simulink model "Vehicle_Light"  (R2022b)
settings: Solver=FixedStepAuto  StartTime=0.0  StopTime=100  RelTol=1e-3
model workspace (MAT data in the model file):
  Auto = Simulink.Parameter
  Auto.Value = 1
  Auto.DataType = 'auto'
  Auto.Complexity = 'real'
  Auto.Dimensions = [1 1]
  BehindVehicleDtct = Simulink.Parameter
  BehindVehicleDtct.Value = 3
  BehindVehicleDtct.DataType = 'auto'
  BehindVehicleDtct.Complexity = 'real'
  BehindVehicleDtct.Dimensions = [1 1]
  BrakeLightOff = Simulink.Parameter
  BrakeLightOff.Value = 0
  BrakeLightOff.DataType = 'auto'
  BrakeLightOff.Complexity = 'real'
  BrakeLightOff.Dimensions = [1 1]
  BrakeLightOn = Simulink.Parameter
  BrakeLightOn.Value = 1
  BrakeLightOn.DataType = 'auto'
  BrakeLightOn.Complexity = 'real'
  BrakeLightOn.Dimensions = [1 1]
  BrokeDownPosition = Simulink.Parameter
  BrokeDownPosition.Value = 1
  BrokeDownPosition.DataType = 'auto'
  BrokeDownPosition.Complexity = 'real'
  BrokeDownPosition.Dimensions = [1 1]
  DoorClose = Simulink.Parameter
  DoorClose.Value = 0
  DoorClose.DataType = 'auto'
  DoorClose.Complexity = 'real'
  DoorClose.Dimensions = [1 1]
  DoorOpen = Simulink.Parameter
  DoorOpen.Value = 1
  DoorOpen.DataType = 'auto'
  DoorOpen.Complexity = 'real'
  DoorOpen.Dimensions = [1 1]
  EscortLightOff = Simulink.Parameter
  EscortLightOff.Value = 0
  EscortLightOff.DataType = 'auto'
  EscortLightOff.Complexity = 'real'
  EscortLightOff.Dimensions = [1 1]
  EscortLightOn = Simulink.Parameter
  EscortLightOn.Value = 1
  EscortLightOn.DataType = 'auto'
  EscortLightOn.Complexity = 'real'
  EscortLightOn.Dimensions = [1 1]
  FogDetect = Simulink.Parameter
  FogDetect.Value = 0
  FogDetect.DataType = 'auto'
  FogDetect.Complexity = 'real'
  FogDetect.Dimensions = [1 1]
  HazardLightOff = Simulink.Parameter
  HazardLightOff.Value = 0
  HazardLightOff.DataType = 'auto'
  HazardLightOff.Complexity = 'real'
  HazardLightOff.Dimensions = [1 1]
  HazardLightOn = Simulink.Parameter
  HazardLightOn.Value = 1
  HazardLightOn.DataType = 'auto'
  HazardLightOn.Complexity = 'real'
  HazardLightOn.Dimensions = [1 1]
  HeadLightOff = Simulink.Parameter
  HeadLightOff.Value = 0
  HeadLightOff.DataType = 'auto'
  HeadLightOff.Complexity = 'real'
  HeadLightOff.Dimensions = [1 1]
  HeadLightOn = Simulink.Parameter
  HeadLightOn.Value = 1
  HeadLightOn.DataType = 'auto'
  HeadLightOn.Complexity = 'real'
  HeadLightOn.Dimensions = [1 1]
  HighBeam = Simulink.Parameter
  HighBeam.Value = 2
  HighBeam.DataType = 'auto'
  HighBeam.Complexity = 'real'
  HighBeam.Dimensions = [1 1]
  Highway = Simulink.Parameter
  Highway.Value = 1
  Highway.DataType = 'auto'
  Highway.Complexity = 'real'
  Highway.Dimensions = [1 1]
  Ignition_OFF = Simulink.Parameter
  Ignition_OFF.Value = 0
  Ignition_OFF.DataType = 'auto'
  Ignition_OFF.Complexity = 'real'
  Ignition_OFF.Dimensions = [1 1]
  Ignition_ON = Simulink.Parameter
  Ignition_ON.Value = 1
  Ignition_ON.DataType = 'auto'
  Ignition_ON.Complexity = 'real'
  Ignition_ON.Dimensions = [1 1]
  InsideCity = Simulink.Parameter
  InsideCity.Value = 4
  InsideCity.DataType = 'auto'
  InsideCity.Complexity = 'real'
  InsideCity.Dimensions = [1 1]
  LeftIndicator = Simulink.Parameter
  LeftIndicator.Value = 2
  LeftIndicator.DataType = 'auto'
  LeftIndicator.Complexity = 'real'
  LeftIndicator.Dimensions = [1 1]
  LeftSideAngle = Simulink.Parameter
  LeftSideAngle.Value = -10
  LeftSideAngle.DataType = 'auto'
  LeftSideAngle.Complexity = 'real'
  LeftSideAngle.Dimensions = [1 1]
  LowBeam = Simulink.Parameter
  LowBeam.Value = 3
  LowBeam.DataType = 'auto'
  LowBeam.Complexity = 'real'
  LowBeam.Dimensions = [1 1]
  LuggageCompartmentClose = Simulink.Parameter
  LuggageCompartmentClose.Value = 0
  LuggageCompartmentClose.DataType = 'auto'
  LuggageCompartmentClose.Complexity = 'real'
  LuggageCompartmentClose.Dimensions = [1 1]
  LuggageCompartmentOpen = Simulink.Parameter
  LuggageCompartmentOpen.Value = 1
  LuggageCompartmentOpen.DataType = 'auto'
  LuggageCompartmentOpen.Complexity = 'real'
  LuggageCompartmentOpen.Dimensions = [1 1]
  Manual = Simulink.Parameter
  Manual.Value = 0
  Manual.DataType = 'auto'
  Manual.Complexity = 'real'
  Manual.Dimensions = [1 1]
  NoVehicleDtct = Simulink.Parameter
  NoVehicleDtct.Value = 0
  NoVehicleDtct.DataType = 'auto'
  NoVehicleDtct.Complexity = 'real'
  NoVehicleDtct.Dimensions = [1 1]
  OnComingVehicle = Simulink.Parameter
  OnComingVehicle.Value = 2
  OnComingVehicle.DataType = 'auto'
  OnComingVehicle.Complexity = 'real'
  OnComingVehicle.Dimensions = [1 1]
  OutsideCity = Simulink.Parameter
  OutsideCity.Value = 2
  OutsideCity.DataType = 'auto'
  OutsideCity.Complexity = 'real'
  OutsideCity.Dimensions = [1 1]
  RainDetect = Simulink.Parameter
  RainDetect.Value = 1
  RainDetect.DataType = 'auto'
  RainDetect.Complexity = 'real'
  RainDetect.Dimensions = [1 1]
  ReadingLightOff = Simulink.Parameter
  ReadingLightOff.Value = 0
  ReadingLightOff.DataType = 'auto'
  ReadingLightOff.Complexity = 'real'
  ReadingLightOff.Dimensions = [1 1]
  ReadingLightOn = Simulink.Parameter
  ReadingLightOn.Value = 1
  ReadingLightOn.DataType = 'auto'
  ReadingLightOn.Complexity = 'real'
  ReadingLightOn.Dimensions = [1 1]
  RightIndicator = Simulink.Parameter
  RightIndicator.Value = 1
  RightIndicator.DataType = 'auto'
  RightIndicator.Complexity = 'real'
  RightIndicator.Dimensions = [1 1]
  RightSideAngle = Simulink.Parameter
  RightSideAngle.Value = 10
  RightSideAngle.DataType = 'auto'
  RightSideAngle.Complexity = 'real'
  RightSideAngle.Dimensions = [1 1]
  SpdLmt = Simulink.Parameter
  SpdLmt.Value = 40
  SpdLmt.DataType = 'auto'
  SpdLmt.Complexity = 'real'
  SpdLmt.Dimensions = [1 1]
  StationaryPosition = Simulink.Parameter
  StationaryPosition.Value = 0
  StationaryPosition.DataType = 'auto'
  StationaryPosition.Complexity = 'real'
  StationaryPosition.Dimensions = [1 1]
  TailLightOff = Simulink.Parameter
  TailLightOff.Value = 3
  TailLightOff.DataType = 'auto'
  TailLightOff.Complexity = 'real'
  TailLightOff.Dimensions = [1 1]
  TailLightOn = Simulink.Parameter
  TailLightOn.Value = 2
  TailLightOn.DataType = 'auto'
  TailLightOn.Complexity = 'real'
  TailLightOn.Dimensions = [1 1]
  Tunnel = Simulink.Parameter
  Tunnel.Value = 3
  Tunnel.DataType = 'auto'
  Tunnel.Complexity = 'real'
  Tunnel.Dimensions = [1 1]
  VehicleDtct = Simulink.Parameter
  VehicleDtct.Value = 1
  VehicleDtct.DataType = 'auto'
  VehicleDtct.Complexity = 'real'
  VehicleDtct.Dimensions = [1 1]
  VehicleLck = Simulink.Parameter
  VehicleLck.Value = 1
  VehicleLck.DataType = 'auto'
  VehicleLck.Complexity = 'real'
  VehicleLck.Dimensions = [1 1]
  VehicleSpd = Simulink.Parameter
  VehicleSpd.Value = 80
  VehicleSpd.DataType = 'auto'
  VehicleSpd.Complexity = 'real'
  VehicleSpd.Dimensions = [1 1]
  VehicleUnlck = Simulink.Parameter
  VehicleUnlck.Value = 0
  VehicleUnlck.DataType = 'auto'
  VehicleUnlck.Complexity = 'real'
  VehicleUnlck.Dimensions = [1 1]
undefined symbols (not defined in the file): BehindVeh_Detect, Fog_Detect, LightSystem, NoVeh_Detect, Rain_Detect, VehicleSpeed
libraries: simulink x74
settings Model: DataDictionary=test.sldd  Creator=sanke  LastModifiedBy=Shaileja Swami
settings DebuggingCC: ParameterPrecisionLossMsg=none  UnconnectedInputMsg=warning  UnconnectedOutputMsg=warning  UnconnectedLineMsg=warning
settings ModelReferenceCC: EnableRefExpFcnMdlSchedulingChecks=on
settings RTWCC: DLArmComputeVersion=19.05

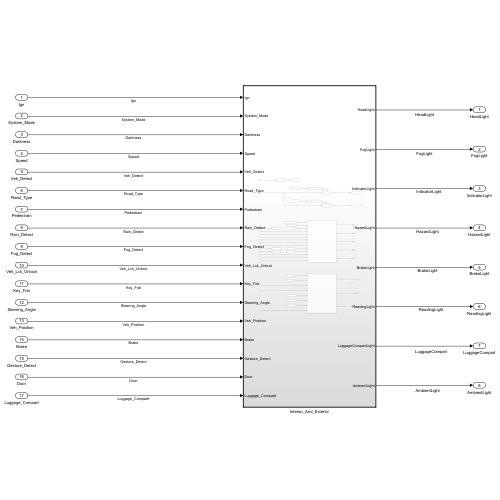
[thumbnail: Simulink's stored preview of the top-level diagram]
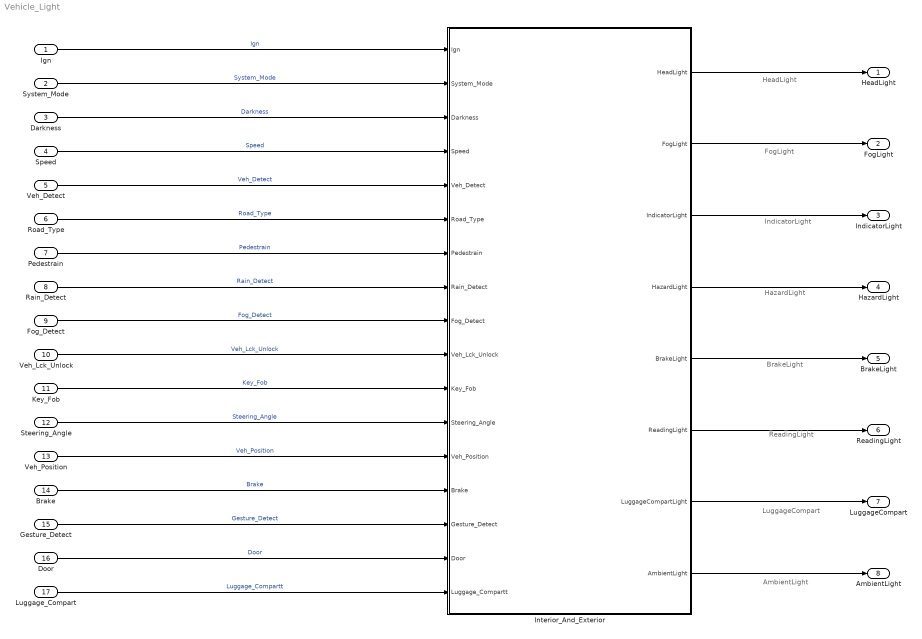
== system Vehicle_Light ==
  note: AmbientLight
  note: LuggageCompart
  note: ReadingLight
  note: BrakeLight
  note: HazardLight
  note: IndicatorLight
  note: FogLight
  note: HeadLight
  Ign : Inport
  System_Mode : Inport  Port=2
  Darkness : Inport  Port=3
  Speed : Inport  Port=4
  Veh_Detect : Inport  Port=5
  Road_Type : Inport  Port=6
  Pedestrain : Inport  Port=7
  Rain_Detect : Inport  Port=8
  Fog_Detect : Inport  Port=9
  Veh_Lck_Unlock : Inport  Port=10
  Key_Fob : Inport  Port=11
  Steering_Angle : Inport  Port=12
  Veh_Position : Inport  Port=13
  Brake : Inport  Port=14
  Gesture_Detect : Inport  Port=15
  Door : Inport  Port=16
  Luggage_Compart : Inport  Port=17
  Interior_And_Exterior : Subsystem  TreatAsAtomicUnit=on
  HeadLight : Outport
  FogLight : Outport  Port=2
  IndicatorLight : Outport  Port=3
  HazardLight : Outport  Port=4
  BrakeLight : Outport  Port=5
  ReadingLight : Outport  Port=6
  LuggageCompart : Outport  Port=7
  AmbientLight : Outport  Port=8
  wires:
  Ign/1 -> Interior_And_Exterior/1(Ign)  "Ign"
  Veh_Detect/1 -> Interior_And_Exterior/5(Veh_Detect)  "Veh_Detect"
  Brake/1 -> Interior_And_Exterior/14(Brake)  "Brake"
  Key_Fob/1 -> Interior_And_Exterior/11(Key_Fob)  "Key_Fob"
  Fog_Detect/1 -> Interior_And_Exterior/9(Fog_Detect)  "Fog_Detect"
  Interior_And_Exterior/8(AmbientLight) -> AmbientLight/1
  Steering_Angle/1 -> Interior_And_Exterior/12(Steering_Angle)  "Steering_Angle"
  Road_Type/1 -> Interior_And_Exterior/6(Road_Type)  "Road_Type"
  Speed/1 -> Interior_And_Exterior/4(Speed)  "Speed"
  Interior_And_Exterior/4(HazardLight) -> HazardLight/1
  Pedestrain/1 -> Interior_And_Exterior/7(Pedestrain)  "Pedestrain"
  Rain_Detect/1 -> Interior_And_Exterior/8(Rain_Detect)  "Rain_Detect"
  Veh_Lck_Unlock/1 -> Interior_And_Exterior/10(Veh_Lck_Unlock)  "Veh_Lck_Unlock"
  Luggage_Compart/1 -> Interior_And_Exterior/17(Luggage_Compartt)  "Luggage_Compartt"
  System_Mode/1 -> Interior_And_Exterior/2(System_Mode)  "System_Mode"
  Interior_And_Exterior/5(BrakeLight) -> BrakeLight/1
  Interior_And_Exterior/2(FogLight) -> FogLight/1
  Interior_And_Exterior/6(ReadingLight) -> ReadingLight/1
  Veh_Position/1 -> Interior_And_Exterior/13(Veh_Position)  "Veh_Position"
  Door/1 -> Interior_And_Exterior/16(Door)  "Door"
  Interior_And_Exterior/7(LuggageCompartLight) -> LuggageCompart/1
  Interior_And_Exterior/1(HeadLight) -> HeadLight/1
  Darkness/1 -> Interior_And_Exterior/3(Darkness)  "Darkness"
  Interior_And_Exterior/3(IndicatorLight) -> IndicatorLight/1
  Gesture_Detect/1 -> Interior_And_Exterior/15(Gesture_Detect)  "Gesture_Detect"

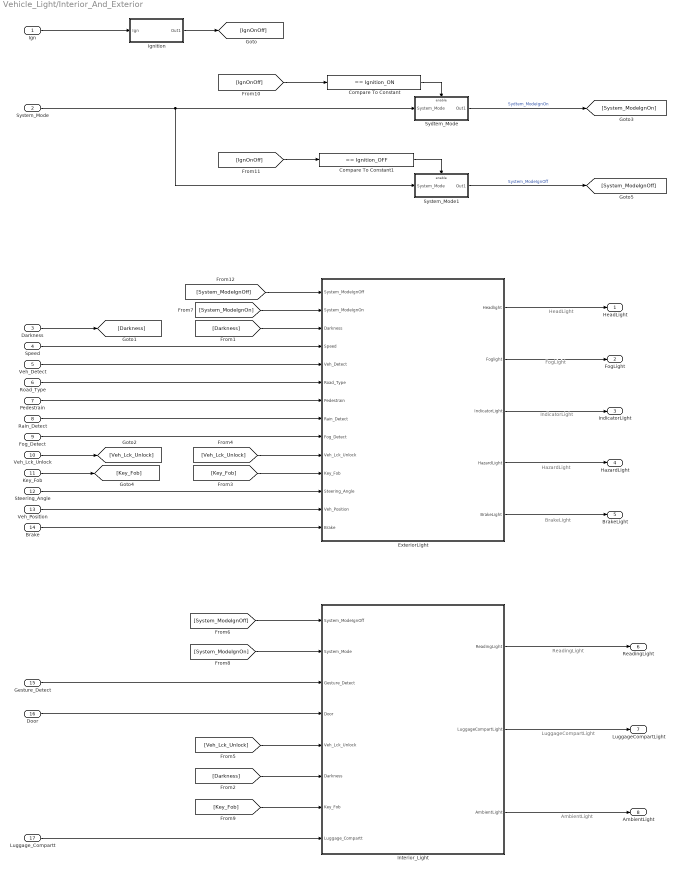
== system Vehicle_Light/Interior_And_Exterior ==
  note: HeadLight
  note: FogLight
  note: IndicatorLight
  note: HazardLight
  note: BrakeLight
  note: ReadingLight
  note: LuggageCompartLight
  note: AmbientLight
  Ign : Inport
  System_Mode : Inport  Port=2
  Darkness : Inport  Port=3
  Speed : Inport  Port=4
  Veh_Detect : Inport  Port=5
  Road_Type : Inport  Port=6
  Pedestrain : Inport  Port=7
  Rain_Detect : Inport  Port=8
  Fog_Detect : Inport  Port=9
  Veh_Lck_Unlock : Inport  Port=10
  Key_Fob : Inport  Port=11
  Steering_Angle : Inport  Port=12
  Veh_Position : Inport  Port=13
  Brake : Inport  Port=14
  Gesture_Detect : Inport  Port=15
  Door : Inport  Port=16
  Luggage_Compartt : Inport  Port=17
  Compare To Constant : simulink/Logic and Bit Operations/Compare To Constant  relop===  const=Ignition_ON  OutDataTypeStr=boolean
  Compare To Constant1 : simulink/Logic and Bit Operations/Compare To Constant  relop===  const=Ignition_OFF  OutDataTypeStr=boolean
  ExteriorLight : Subsystem  TreatAsAtomicUnit=on
  Ignition : Subsystem  TreatAsAtomicUnit=on
  Interior_Light : Subsystem  TreatAsAtomicUnit=on
  Sydtem_Mode : Subsystem  TreatAsAtomicUnit=on
  System_Mode1 : Subsystem  TreatAsAtomicUnit=on
  HeadLight : Outport
  FogLight : Outport  Port=2
  IndicatorLight : Outport  Port=3
  HazardLight : Outport  Port=4
  BrakeLight : Outport  Port=5
  ReadingLight : Outport  Port=6
  LuggageCompartLight : Outport  Port=7
  AmbientLight : Outport  Port=8
  wires:
  Ign/1 -> Ignition/1(Ign)
  System_Mode/1 -> Sydtem_Mode/1(System_Mode), System_Mode1/1(System_Mode)
  Ignition/1(Out1) -> [IgnOnOff]
  [System_ModeIgnOff] -> ExteriorLight/1(System_ModeIgnOff)
  Speed/1 -> ExteriorLight/4(Speed)
  Veh_Detect/1 -> ExteriorLight/5(Veh_Detect)
  Road_Type/1 -> ExteriorLight/6(Road_Type)
  Pedestrain/1 -> ExteriorLight/7(Pedestrain)
  Rain_Detect/1 -> ExteriorLight/8(Rain_Detect)
  Fog_Detect/1 -> ExteriorLight/9(Fog_Detect)
  Steering_Angle/1 -> ExteriorLight/12(Steering_Angle)
  Veh_Position/1 -> ExteriorLight/13(Veh_Position)
  Brake/1 -> ExteriorLight/14(Brake)
  ExteriorLight/1(Headlight) -> HeadLight/1
  ExteriorLight/2(Foglight) -> FogLight/1
  ExteriorLight/3(IndicatorLight) -> IndicatorLight/1
  ExteriorLight/4(HazardLight) -> HazardLight/1
  ExteriorLight/5(BrakeLight) -> BrakeLight/1
  Gesture_Detect/1 -> Interior_Light/3(Gesture_Detect)
  Door/1 -> Interior_Light/4(Door)
  Luggage_Compartt/1 -> Interior_Light/8(Luggage_Compartt)
  Darkness/1 -> [Darkness]
  [Darkness] -> ExteriorLight/3(Darkness)
  [Darkness] -> Interior_Light/6(Darkness)
  Veh_Lck_Unlock/1 -> [Veh_Lck_Unlock]
  [Veh_Lck_Unlock] -> ExteriorLight/10(Veh_Lck_Unlock)
  [Veh_Lck_Unlock] -> Interior_Light/5(Veh_Lck_Unlock)
  Interior_Light/1(ReadingLight) -> ReadingLight/1
  Interior_Light/2(LuggageCompartLight) -> LuggageCompartLight/1
  [System_ModeIgnOff] -> Interior_Light/1(System_ModeIgnOff)
  Sydtem_Mode/1(Out1) -> [System_ModeIgnOn]  "Sydtem_ModeIgnOn"
  [System_ModeIgnOn] -> ExteriorLight/2(System_ModeIgnOn)
  [System_ModeIgnOn] -> Interior_Light/2(System_Mode)
  Interior_Light/3(AmbientLight) -> AmbientLight/1
  Key_Fob/1 -> [Key_Fob]
  [Key_Fob] -> ExteriorLight/11(Key_Fob)
  [Key_Fob] -> Interior_Light/7(Key_Fob)
  [IgnOnOff] -> Compare To Constant/1
  [IgnOnOff] -> Compare To Constant1/1
  Compare To Constant/1 -> Sydtem_Mode/Enable
  Compare To Constant1/1 -> System_Mode1/Enable
  System_Mode1/1(Out1) -> [System_ModeIgnOff]  "System_ModeIgnOff"

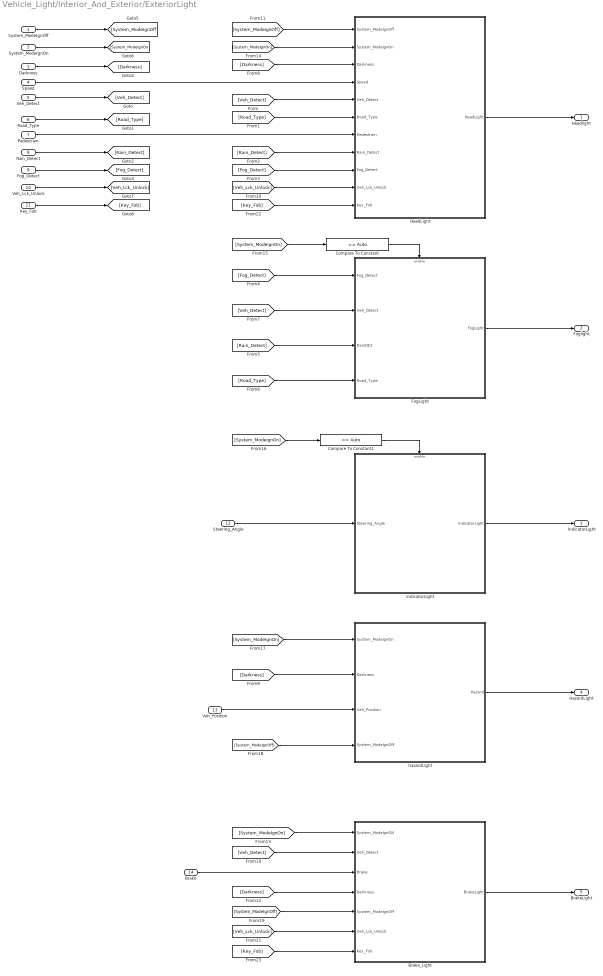
== system Vehicle_Light/Interior_And_Exterior/ExteriorLight ==
  System_ModeIgnOff : Inport
  System_ModeIgnOn : Inport  Port=2
  Darkness : Inport  Port=3
  Speed : Inport  Port=4
  Veh_Detect : Inport  Port=5
  Road_Type : Inport  Port=6
  Pedestrain : Inport  Port=7
  Rain_Detect : Inport  Port=8
  Fog_Detect : Inport  Port=9
  Veh_Lck_Unlock : Inport  Port=10
  Key_Fob : Inport  Port=11
  Steering_Angle : Inport  Port=12
  Veh_Position : Inport  Port=13
  Brake : Inport  Port=14
  Brake_Light : Subsystem  TreatAsAtomicUnit=on
  Compare To Constant : simulink/Logic and Bit Operations/Compare To Constant  relop===  const=Auto  OutDataTypeStr=boolean
  Compare To Constant1 : simulink/Logic and Bit Operations/Compare To Constant  relop===  const=Auto  OutDataTypeStr=boolean
  FogLight : Subsystem  TreatAsAtomicUnit=on
  HeadLight : Subsystem  TreatAsAtomicUnit=on
  hazardLight : Subsystem  TreatAsAtomicUnit=on
  indicatorLight : Subsystem  TreatAsAtomicUnit=on
  Headlight : Outport
  Foglight : Outport  Port=2
  IndicatorLight : Outport  Port=3
  HazardLight : Outport  Port=4
  BrakeLight : Outport  Port=5
  wires:
  Speed/1 -> HeadLight/4(Speed)
  Pedestrain/1 -> HeadLight/7(Pedestrain)
  Veh_Detect/1 -> [Veh_Detect]
  Road_Type/1 -> [Road_Type]
  Rain_Detect/1 -> [Rain_Detect]
  Fog_Detect/1 -> [Fog_Detect]
  [Veh_Detect] -> HeadLight/5(Veh_Detect)
  [Road_Type] -> HeadLight/6(Road_Type)
  [Rain_Detect] -> HeadLight/8(Rain_Detect)
  [Fog_Detect] -> HeadLight/9(Fog_Detect)
  [Fog_Detect] -> FogLight/1(Fog_Detect)
  [Rain_Detect] -> FogLight/3(RainDtct)
  [Road_Type] -> FogLight/4(Road_Type)
  [Veh_Detect] -> FogLight/2(Veh_Detect)
  Steering_Angle/1 -> indicatorLight/1(Steering_Angle)
  Darkness/1 -> [Darkness]
  [Darkness] -> HeadLight/3(Darkness)
  [Darkness] -> hazardLight/2(Darkness)
  Veh_Position/1 -> hazardLight/3(Veh_Position)
  [Veh_Detect] -> Brake_Light/2(Veh_Detect)
  Brake/1 -> Brake_Light/3(Brake)
  FogLight/1(FogLight) -> Foglight/1
  indicatorLight/1(IndicatorLight) -> IndicatorLight/1
  [Darkness] -> Brake_Light/4(Darkness)
  System_ModeIgnOff/1 -> [System_ModeIgnOff]
  [System_ModeIgnOff] -> HeadLight/1(System_ModeIgnOff)
  [System_ModeIgnOff] -> Brake_Light/5(System_ModeIgnOff)
  HeadLight/1(HeadLight) -> Headlight/1
  System_ModeIgnOn/1 -> [System_ModeIgnOn]
  [System_ModeIgnOn] -> HeadLight/2(System_ModeIgnOn)
  [System_ModeIgnOn] -> Compare To Constant/1
  Compare To Constant/1 -> FogLight/Enable
  [System_ModeIgnOn] -> Compare To Constant1/1
  Compare To Constant1/1 -> indicatorLight/Enable
  [System_ModeIgnOff] -> hazardLight/4(System_ModeIgnOff)
  [System_ModeIgnOn] -> hazardLight/1(System_ModeIgnOn)
  hazardLight/1(Hazard) -> HazardLight/1
  [System_ModeIgnOn] -> Brake_Light/1(System_ModeIgnON)
  Veh_Lck_Unlock/1 -> [Veh_Lck_Unlock]
  [Veh_Lck_Unlock] -> HeadLight/10(Veh_Lck_Unlock)
  [Veh_Lck_Unlock] -> Brake_Light/6(Veh_Lck_Unlock)
  Key_Fob/1 -> [Key_Fob]
  [Key_Fob] -> HeadLight/11(Key_Fob)
  [Key_Fob] -> Brake_Light/7(Key_Fob)
  Brake_Light/1(BrakeLight) -> BrakeLight/1

== system Vehicle_Light/Interior_And_Exterior/Ignition ==
  Ign : Inport
  Constant : Constant  Value=Ignition_ON  SampleTime=-1
  Constant1 : Constant  Value=Ignition_OFF  SampleTime=-1
  Switch : Switch  Criteria=u2 > Threshold  SaturateOnIntegerOverflow=off  InputSameDT=off
  Out1 : Outport
  wires:
  Ign/1 -> Switch/2
  Switch/1 -> Out1/1
  Constant/1 -> Switch/1
  Constant1/1 -> Switch/3

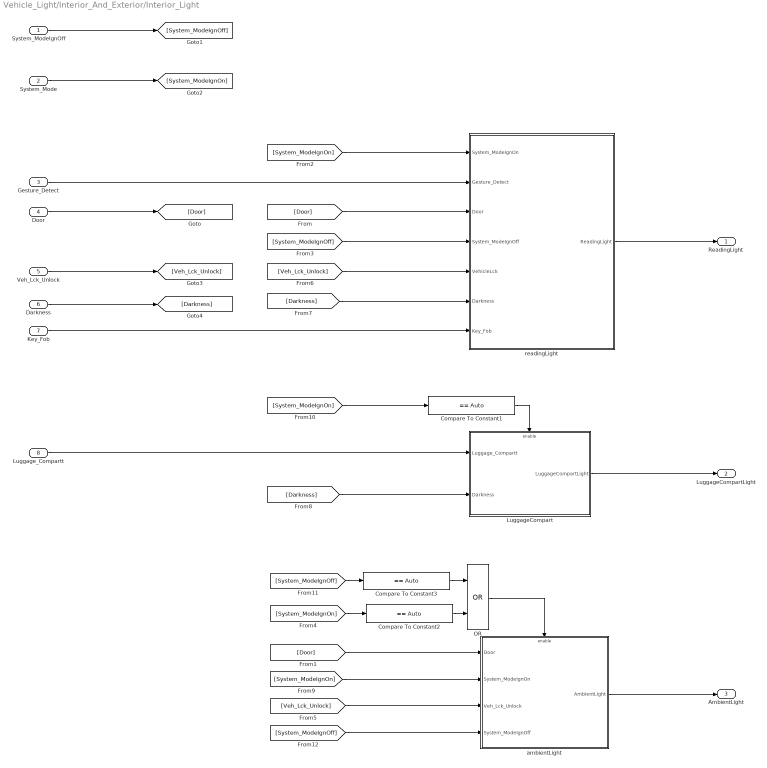
== system Vehicle_Light/Interior_And_Exterior/Interior_Light ==
  System_ModeIgnOff : Inport
  System_Mode : Inport  Port=2
  Gesture_Detect : Inport  Port=3
  Door : Inport  Port=4
  Veh_Lck_Unlock : Inport  Port=5
  Darkness : Inport  Port=6
  Key_Fob : Inport  Port=7
  Luggage_Compartt : Inport  Port=8
  Compare To Constant1 : simulink/Logic and Bit Operations/Compare To Constant  relop===  const=Auto  OutDataTypeStr=boolean
  Compare To Constant2 : simulink/Logic and Bit Operations/Compare To Constant  relop===  const=Auto  OutDataTypeStr=boolean
  Compare To Constant3 : simulink/Logic and Bit Operations/Compare To Constant  relop===  const=Auto  OutDataTypeStr=boolean
  LuggageCompart : Subsystem  TreatAsAtomicUnit=on
  OR : Logic  Operator=OR  AllPortsSameDT=off  OutDataTypeStr=boolean
  ambientLight : Subsystem  TreatAsAtomicUnit=on
  readingLight : Subsystem  TreatAsAtomicUnit=on
  ReadingLight : Outport
  LuggageCompartLight : Outport  Port=2
  AmbientLight : Outport  Port=3
  wires:
  Gesture_Detect/1 -> readingLight/2(Gesture_Detect)
  Luggage_Compartt/1 -> LuggageCompart/1(Luggage_Compartt)
  LuggageCompart/1(LuggageCompartLight) -> LuggageCompartLight/1
  Door/1 -> [Door]
  [Door] -> readingLight/3(Door)
  [Door] -> ambientLight/1(Door)
  ambientLight/1(AmbientLight) -> AmbientLight/1
  System_ModeIgnOff/1 -> [System_ModeIgnOff]
  [System_ModeIgnOn] -> readingLight/1(System_ModeIgnOn)
  [System_ModeIgnOff] -> readingLight/4(System_ModeIgnOff)
  Veh_Lck_Unlock/1 -> [Veh_Lck_Unlock]
  [Veh_Lck_Unlock] -> ambientLight/3(Veh_Lck_Unlock)
  [Veh_Lck_Unlock] -> readingLight/5(VehicleLck)
  Darkness/1 -> [Darkness]
  [Darkness] -> readingLight/6(Darkness)
  [Darkness] -> LuggageCompart/2(Darkness)
  [System_ModeIgnOn] -> ambientLight/2(System_ModeIgnOn)
  Compare To Constant1/1 -> LuggageCompart/Enable
  [System_ModeIgnOn] -> Compare To Constant1/1
  Key_Fob/1 -> readingLight/7(Key_Fob)
  System_Mode/1 -> [System_ModeIgnOn]
  [System_ModeIgnOn] -> Compare To Constant2/1
  readingLight/1(ReadingLight) -> ReadingLight/1
  [System_ModeIgnOff] -> Compare To Constant3/1
  Compare To Constant3/1 -> OR/1
  Compare To Constant2/1 -> OR/2
  OR/1 -> ambientLight/Enable
  [System_ModeIgnOff] -> ambientLight/4(System_ModeIgnOff)

== system Vehicle_Light/Interior_And_Exterior/Sydtem_Mode ==
  System_Mode : Inport
  Enable : EnablePort
  Constant : Constant  Value=Auto  SampleTime=-1
  Constant1 : Constant  Value=Manual  SampleTime=-1
  Switch : Switch  Criteria=u2 > Threshold  SaturateOnIntegerOverflow=off  InputSameDT=off
  Out1 : Outport
  wires:
  Switch/1 -> Out1/1
  System_Mode/1 -> Switch/2
  Constant/1 -> Switch/1
  Constant1/1 -> Switch/3

== system Vehicle_Light/Interior_And_Exterior/System_Mode1 ==
  System_Mode : Inport
  Enable : EnablePort
  Constant : Constant  Value=Auto  SampleTime=-1
  Constant1 : Constant  Value=Manual  SampleTime=-1
  Switch : Switch  Criteria=u2 > Threshold  SaturateOnIntegerOverflow=off  InputSameDT=off
  Out1 : Outport
  wires:
  Constant1/1 -> Switch/3
  Constant/1 -> Switch/1
  System_Mode/1 -> Switch/2
  Switch/1 -> Out1/1

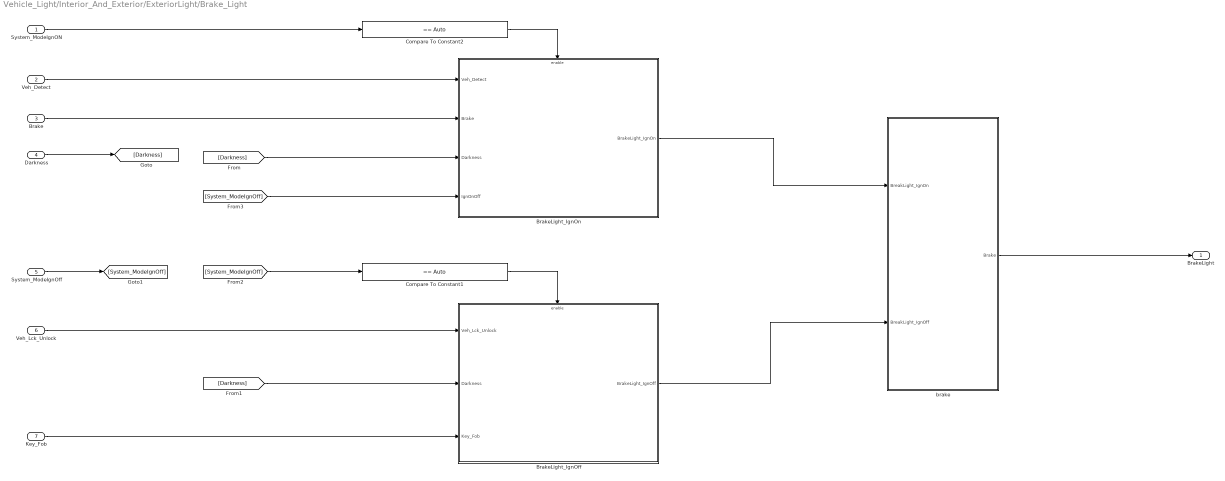
== system Vehicle_Light/Interior_And_Exterior/ExteriorLight/Brake_Light ==
  System_ModeIgnON : Inport
  Veh_Detect : Inport  Port=2
  Brake : Inport  Port=3
  Darkness : Inport  Port=4
  System_ModeIgnOff : Inport  Port=5
  Veh_Lck_Unlock : Inport  Port=6
  Key_Fob : Inport  Port=7
  BrakeLight_IgnOff : Subsystem
  BrakeLight_IgnOn : Subsystem
  Compare To Constant1 : simulink/Logic and Bit Operations/Compare To Constant  relop===  const=Auto  OutDataTypeStr=boolean
  Compare To Constant2 : simulink/Logic and Bit Operations/Compare To Constant  relop===  const=Auto  OutDataTypeStr=boolean
  brake : Subsystem
  BrakeLight : Outport
  wires:
  Veh_Detect/1 -> BrakeLight_IgnOn/1(Veh_Detect)
  Brake/1 -> BrakeLight_IgnOn/2(Brake)
  Darkness/1 -> [Darkness]
  [Darkness] -> BrakeLight_IgnOn/3(Darkness)
  [Darkness] -> BrakeLight_IgnOff/2(Darkness)
  Veh_Lck_Unlock/1 -> BrakeLight_IgnOff/1(Veh_Lck_Unlock)
  Key_Fob/1 -> BrakeLight_IgnOff/3(Key_Fob)
  Compare To Constant1/1 -> BrakeLight_IgnOff/Enable
  System_ModeIgnOff/1 -> [System_ModeIgnOff]
  [System_ModeIgnOff] -> Compare To Constant1/1
  [System_ModeIgnOff] -> BrakeLight_IgnOn/4(IgnOnOff)
  Compare To Constant2/1 -> BrakeLight_IgnOn/Enable
  System_ModeIgnON/1 -> Compare To Constant2/1
  BrakeLight_IgnOff/1(BrakeLight_IgnOff) -> brake/2(BreakLight_IgnOff)
  BrakeLight_IgnOn/1(BrakeLight_IgnOn) -> brake/1(BreakLight_IgnOn)
  brake/1(Brake) -> BrakeLight/1

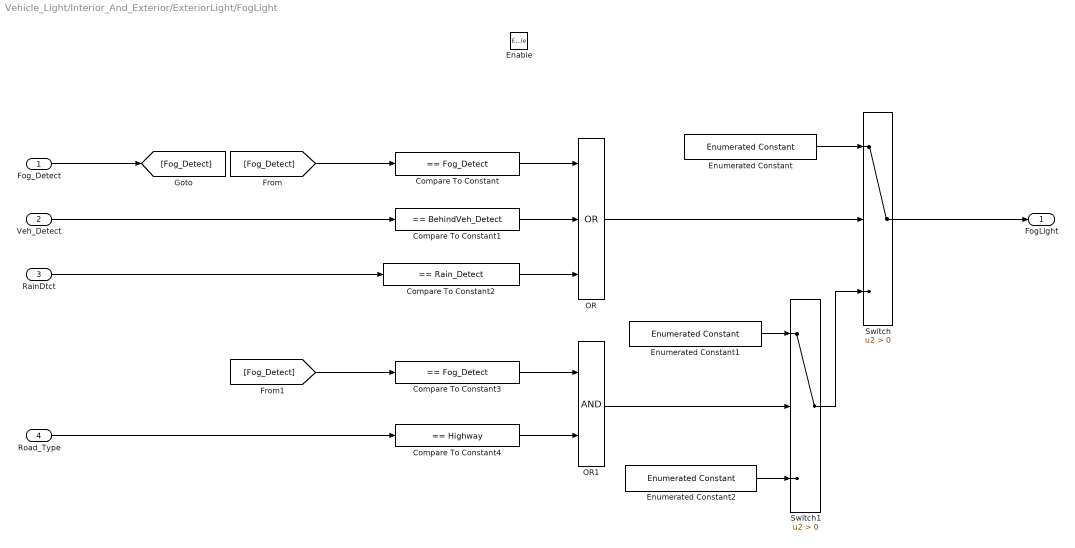
== system Vehicle_Light/Interior_And_Exterior/ExteriorLight/FogLight ==
  Fog_Detect : Inport
  Veh_Detect : Inport  Port=2
  RainDtct : Inport  Port=3
  Road_Type : Inport  Port=4
  Enable : EnablePort
  Compare To Constant : simulink/Logic and Bit Operations/Compare To Constant  relop===  const=Fog_Detect  OutDataTypeStr=boolean
  Compare To Constant1 : simulink/Logic and Bit Operations/Compare To Constant  relop===  const=BehindVeh_Detect  OutDataTypeStr=boolean
  Compare To Constant2 : simulink/Logic and Bit Operations/Compare To Constant  relop===  const=Rain_Detect  OutDataTypeStr=boolean
  Compare To Constant3 : simulink/Logic and Bit Operations/Compare To Constant  relop===  const=Fog_Detect  OutDataTypeStr=boolean
  Compare To Constant4 : simulink/Logic and Bit Operations/Compare To Constant  relop===  const=Highway  OutDataTypeStr=boolean
  Enumerated Constant : simulink/Sources/Enumerated Constant  OutDataTypeStr=Enum: LightSystem  Value=LightSystem.FogLightOn  SampleTime=-1
  Enumerated Constant1 : simulink/Sources/Enumerated Constant  OutDataTypeStr=Enum: LightSystem  Value=LightSystem.FogLightOff  SampleTime=-1
  Enumerated Constant2 : simulink/Sources/Enumerated Constant  OutDataTypeStr=Enum: LightSystem  Value=LightSystem.FogLightOff  SampleTime=-1
  OR : Logic  Operator=OR  Inputs=3  AllPortsSameDT=off  OutDataTypeStr=boolean
  OR1 : Logic  AllPortsSameDT=off  OutDataTypeStr=boolean
  Switch : Switch  Criteria=u2 > Threshold  SaturateOnIntegerOverflow=off  InputSameDT=off
  Switch1 : Switch  Criteria=u2 > Threshold  SaturateOnIntegerOverflow=off  InputSameDT=off
  FogLight : Outport
  wires:
  Switch1/1 -> Switch/3
  OR/1 -> Switch/2
  OR1/1 -> Switch1/2
  Compare To Constant/1 -> OR/1
  Compare To Constant1/1 -> OR/2
  Compare To Constant2/1 -> OR/3
  Compare To Constant3/1 -> OR1/1
  Compare To Constant4/1 -> OR1/2
  Veh_Detect/1 -> Compare To Constant1/1
  RainDtct/1 -> Compare To Constant2/1
  Road_Type/1 -> Compare To Constant4/1
  Fog_Detect/1 -> [Fog_Detect]
  [Fog_Detect] -> Compare To Constant/1
  [Fog_Detect] -> Compare To Constant3/1
  Switch/1 -> FogLight/1
  Enumerated Constant/1 -> Switch/1
  Enumerated Constant1/1 -> Switch1/1
  Enumerated Constant2/1 -> Switch1/3

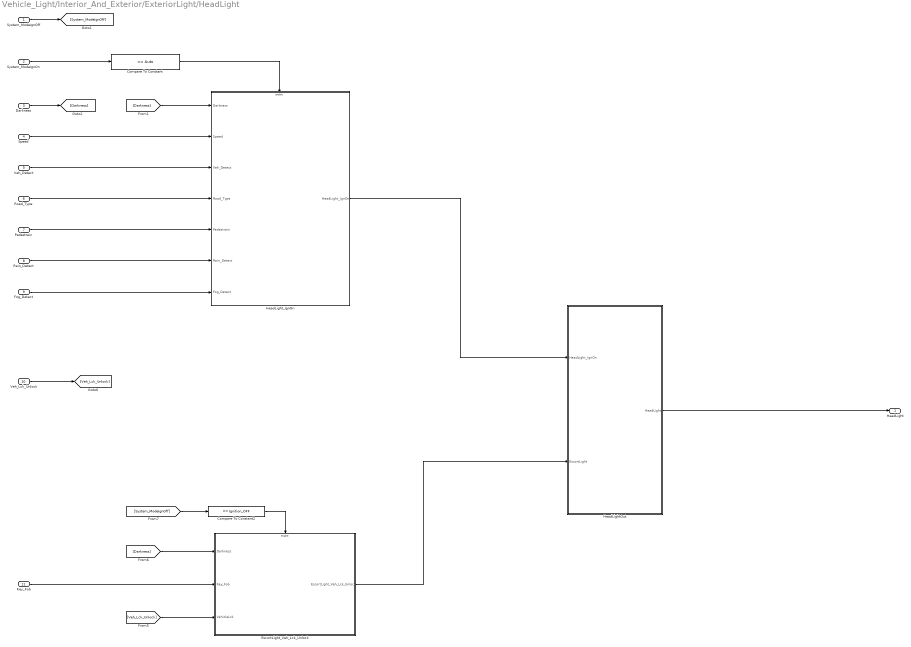
== system Vehicle_Light/Interior_And_Exterior/ExteriorLight/HeadLight ==
  System_ModeIgnOff : Inport
  System_ModeIgnOn : Inport  Port=2
  Darkness : Inport  Port=3
  Speed : Inport  Port=4
  Veh_Detect : Inport  Port=5
  Road_Type : Inport  Port=6
  Pedestrain : Inport  Port=7
  Rain_Detect : Inport  Port=8
  Fog_Detect : Inport  Port=9
  Veh_Lck_Unlock : Inport  Port=10
  Key_Fob : Inport  Port=11
  Compare To Constant : simulink/Logic and Bit Operations/Compare To Constant  relop===  const=Auto  OutDataTypeStr=boolean
  Compare To Constant2 : simulink/Logic and Bit Operations/Compare To Constant  relop===  const=Ignition_OFF  OutDataTypeStr=boolean
  EscortLight_Veh_Lck_Unlock : Subsystem  TreatAsAtomicUnit=on
  HeadLightOut : Subsystem
  HeadLight_IgnOn : Subsystem
  HeadLight : Outport
  wires:
  Veh_Lck_Unlock/1 -> [Veh_Lck_Unlock]
  Speed/1 -> HeadLight_IgnOn/2(Speed)
  Veh_Detect/1 -> HeadLight_IgnOn/3(Veh_Detect)
  Road_Type/1 -> HeadLight_IgnOn/4(Road_Type)
  Pedestrain/1 -> HeadLight_IgnOn/5(Pedestrain)
  Rain_Detect/1 -> HeadLight_IgnOn/6(Rain_Detect)
  Fog_Detect/1 -> HeadLight_IgnOn/7(Fog_Detect)
  HeadLight_IgnOn/1(HeadLight_IgnOn) -> HeadLightOut/1(HeadLight_IgnOn)
  System_ModeIgnOff/1 -> [System_ModeIgnOff]
  Darkness/1 -> [Darkness]
  [Darkness] -> HeadLight_IgnOn/1(Darkness)
  HeadLightOut/1(HeadLight) -> HeadLight/1
  [Veh_Lck_Unlock] -> EscortLight_Veh_Lck_Unlock/3(VehicleLck)
  Key_Fob/1 -> EscortLight_Veh_Lck_Unlock/2(Key_Fob)
  [Darkness] -> EscortLight_Veh_Lck_Unlock/1(Darkness)
  [System_ModeIgnOff] -> Compare To Constant2/1
  Compare To Constant2/1 -> EscortLight_Veh_Lck_Unlock/Enable
  System_ModeIgnOn/1 -> Compare To Constant/1
  Compare To Constant/1 -> HeadLight_IgnOn/Enable
  EscortLight_Veh_Lck_Unlock/1(EscortLight_Veh_Lck_Unlock) -> HeadLightOut/2(EscortLight)

== system Vehicle_Light/Interior_And_Exterior/ExteriorLight/hazardLight ==
  System_ModeIgnOn : Inport
  Darkness : Inport  Port=2
  Veh_Position : Inport  Port=3
  System_ModeIgnOff : Inport  Port=4
  Compare To Constant : simulink/Logic and Bit Operations/Compare To Constant  relop===  const=Auto  OutDataTypeStr=boolean
  Compare To Constant1 : simulink/Logic and Bit Operations/Compare To Constant  relop===  const=Auto  OutDataTypeStr=boolean
  HazardLightIgnOff : Subsystem
  HazardLightIgnOn : Subsystem
  Subsystem : Subsystem
  Hazard : Outport
  wires:
  Darkness/1 -> [Darkness]
  [Darkness] -> HazardLightIgnOn/1(Darkness)
  [Darkness] -> HazardLightIgnOff/1(Darkness)
  Veh_Position/1 -> [Veh_Position]
  [Veh_Position] -> HazardLightIgnOn/2(Veh_Position)
  [Veh_Position] -> HazardLightIgnOff/2(Veh_Position)
  Compare To Constant/1 -> HazardLightIgnOff/Enable
  System_ModeIgnOff/1 -> Compare To Constant/1
  Compare To Constant1/1 -> HazardLightIgnOn/Enable
  System_ModeIgnOn/1 -> Compare To Constant1/1
  HazardLightIgnOn/1(HazardLightOn) -> Subsystem/1(HazardLightIgnOn)
  HazardLightIgnOff/1(HazardLightOff) -> Subsystem/2(HazardLightIgnOff)
  Subsystem/1(Hazard) -> Hazard/1

== system Vehicle_Light/Interior_And_Exterior/ExteriorLight/indicatorLight ==
  Steering_Angle : Inport
  Enable : EnablePort
  Indicator : Stateflow chart  TreatAsAtomicUnit=on
  Subsystem : Subsystem
  IndicatorLight : Outport
  wires:
  Steering_Angle/1 -> Indicator/1(Steering_Angle)
  Indicator/1(Indicator) -> Subsystem/1(IndicatorLight)
  Subsystem/1(IndicatorLightOnOFF) -> IndicatorLight/1

== system Vehicle_Light/Interior_And_Exterior/Interior_Light/LuggageCompart ==
  Luggage_Compartt : Inport
  Darkness : Inport  Port=2
  Enable : EnablePort
  AND : Logic  AllPortsSameDT=off  OutDataTypeStr=boolean
  Enumerated Constant : simulink/Sources/Enumerated Constant  OutDataTypeStr=Enum: LightSystem  Value=LightSystem.LuggageCompartLightOn  SampleTime=-1
  Enumerated Constant1 : simulink/Sources/Enumerated Constant  OutDataTypeStr=Enum: LightSystem  Value=LightSystem.LuggageCompartLightOff  SampleTime=-1
  Switch : Switch  Criteria=u2 > Threshold  SaturateOnIntegerOverflow=off  InputSameDT=off
  LuggageCompartLight : Outport
  wires:
  Luggage_Compartt/1 -> AND/1
  Darkness/1 -> AND/2
  AND/1 -> Switch/2
  Switch/1 -> LuggageCompartLight/1
  Enumerated Constant/1 -> Switch/1
  Enumerated Constant1/1 -> Switch/3

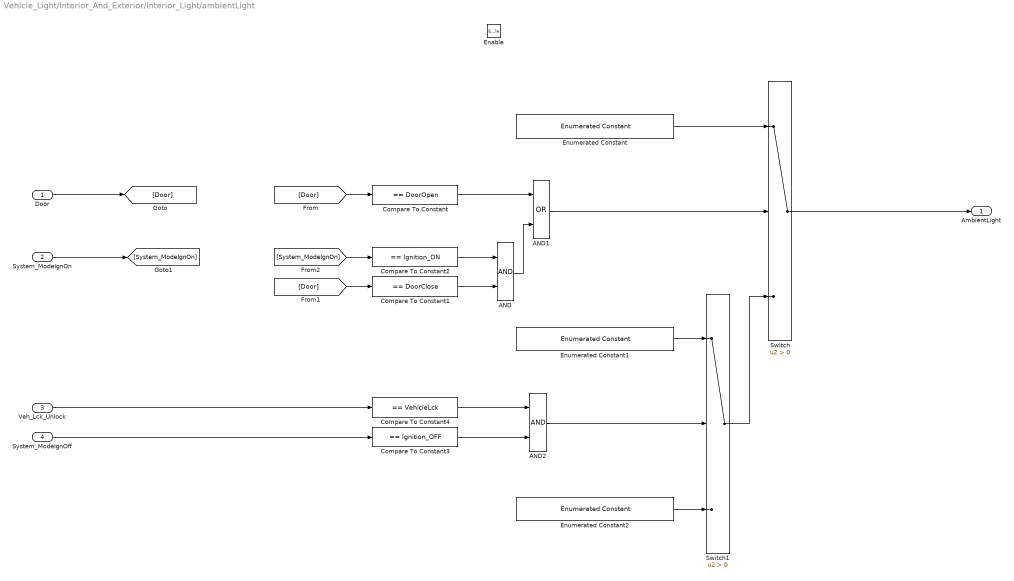
== system Vehicle_Light/Interior_And_Exterior/Interior_Light/ambientLight ==
  Door : Inport
  System_ModeIgnOn : Inport  Port=2
  Veh_Lck_Unlock : Inport  Port=3
  System_ModeIgnOff : Inport  Port=4
  Enable : EnablePort
  AND : Logic  AllPortsSameDT=off  OutDataTypeStr=boolean
  AND1 : Logic  Operator=OR  AllPortsSameDT=off  OutDataTypeStr=boolean
  AND2 : Logic  AllPortsSameDT=off  OutDataTypeStr=boolean
  Compare To Constant : simulink/Logic and Bit Operations/Compare To Constant  relop===  const=DoorOpen  OutDataTypeStr=boolean
  Compare To Constant1 : simulink/Logic and Bit Operations/Compare To Constant  relop===  const=DoorClose  OutDataTypeStr=boolean
  Compare To Constant2 : simulink/Logic and Bit Operations/Compare To Constant  relop===  const=Ignition_ON  OutDataTypeStr=boolean
  Compare To Constant3 : simulink/Logic and Bit Operations/Compare To Constant  relop===  const=Ignition_OFF  OutDataTypeStr=boolean
  Compare To Constant4 : simulink/Logic and Bit Operations/Compare To Constant  relop===  const=VehicleLck  OutDataTypeStr=boolean
  Enumerated Constant : simulink/Sources/Enumerated Constant  OutDataTypeStr=Enum: LightSystem  Value=LightSystem.AmbientLightOn  SampleTime=-1
  Enumerated Constant1 : simulink/Sources/Enumerated Constant  OutDataTypeStr=Enum: LightSystem  Value=LightSystem.AmbientLightOn  SampleTime=-1
  Enumerated Constant2 : simulink/Sources/Enumerated Constant  OutDataTypeStr=Enum: LightSystem  Value=LightSystem.AmbientLightOff  SampleTime=-1
  Switch : Switch  Criteria=u2 > Threshold  SaturateOnIntegerOverflow=off  InputSameDT=off
  Switch1 : Switch  Criteria=u2 > Threshold  SaturateOnIntegerOverflow=off  InputSameDT=off
  AmbientLight : Outport
  wires:
  AND/1 -> AND1/2
  Compare To Constant/1 -> AND1/1
  Door/1 -> [Door]
  [Door] -> Compare To Constant/1
  [Door] -> Compare To Constant1/1
  Compare To Constant1/1 -> AND/2
  Compare To Constant2/1 -> AND/1
  AND1/1 -> Switch/2
  Switch/1 -> AmbientLight/1
  Switch1/1 -> Switch/3
  System_ModeIgnOn/1 -> [System_ModeIgnOn]
  [System_ModeIgnOn] -> Compare To Constant2/1
  AND2/1 -> Switch1/2
  Compare To Constant4/1 -> AND2/1
  Veh_Lck_Unlock/1 -> Compare To Constant4/1
  Compare To Constant3/1 -> AND2/2
  Enumerated Constant/1 -> Switch/1
  Enumerated Constant1/1 -> Switch1/1
  Enumerated Constant2/1 -> Switch1/3
  System_ModeIgnOff/1 -> Compare To Constant3/1

== system Vehicle_Light/Interior_And_Exterior/Interior_Light/readingLight ==
  System_ModeIgnOn : Inport
  Gesture_Detect : Inport  Port=2
  Door : Inport  Port=3
  System_ModeIgnOff : Inport  Port=4
  VehicleLck : Inport  Port=5
  Darkness : Inport  Port=6
  Key_Fob : Inport  Port=7
  Compare To Constant : simulink/Logic and Bit Operations/Compare To Constant  relop===  const=Auto  OutDataTypeStr=boolean
  Compare To Constant1 : simulink/Logic and Bit Operations/Compare To Constant  relop===  const=Auto  OutDataTypeStr=boolean
  Subsystem : Subsystem
  Subsystem1 : Subsystem
  Subsystem2 : Subsystem
  ReadingLight : Outport
  wires:
  Gesture_Detect/1 -> Subsystem/1(Gesture_Detect)
  Door/1 -> Subsystem/2(Door)
  Subsystem/1(ReadingLight_IgnOn) -> Subsystem2/1(ReadingLight_IgnOn)
  System_ModeIgnOn/1 -> Compare To Constant/1
  Compare To Constant/1 -> Subsystem/Enable
  VehicleLck/1 -> Subsystem1/1(VehicleLck)
  Darkness/1 -> Subsystem1/2(Darkness)
  Key_Fob/1 -> Subsystem1/3(Key_Fob)
  System_ModeIgnOff/1 -> Compare To Constant1/1
  Compare To Constant1/1 -> Subsystem1/Enable
  Subsystem1/1(ReadingLight_IgnOff) -> Subsystem2/2(ReadingLight_IgnOff)
  Subsystem2/1(ReadingLight) -> ReadingLight/1

== system Vehicle_Light/Interior_And_Exterior/ExteriorLight/Brake_Light/BrakeLight_IgnOff ==
  Veh_Lck_Unlock : Inport
  Darkness : Inport  Port=2
  Key_Fob : Inport  Port=3
  Enable : EnablePort
  Chart1 : Stateflow chart  TreatAsAtomicUnit=on
  BrakeLight_IgnOff : Outport
  wires:
  Chart1/1(BrakeLight) -> BrakeLight_IgnOff/1
  Veh_Lck_Unlock/1 -> Chart1/1(VehicleLck)
  Darkness/1 -> Chart1/2(Darkness)
  Key_Fob/1 -> Chart1/3(Key_Fob)

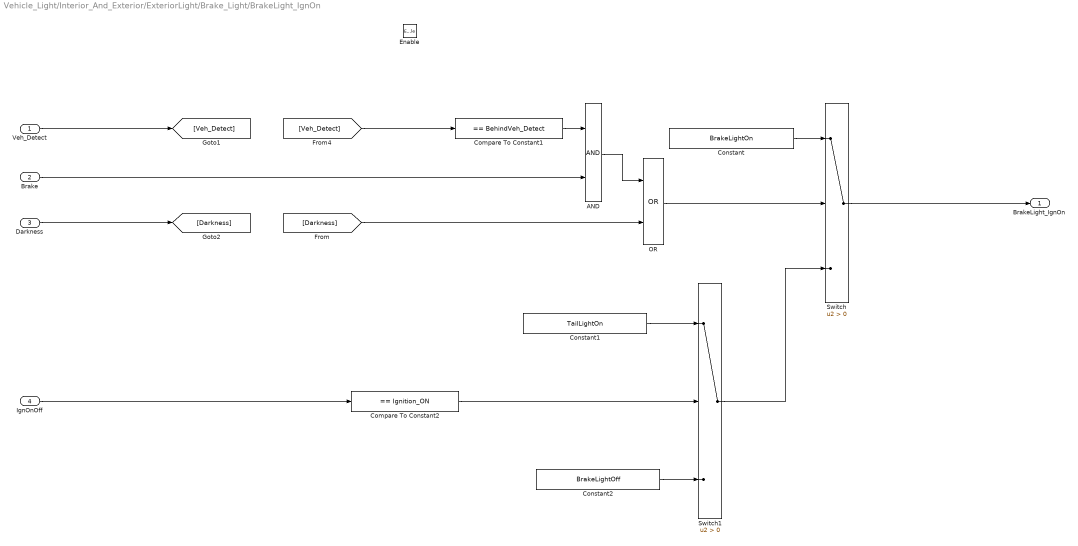
== system Vehicle_Light/Interior_And_Exterior/ExteriorLight/Brake_Light/BrakeLight_IgnOn ==
  Veh_Detect : Inport
  Brake : Inport  Port=2
  Darkness : Inport  Port=3
  IgnOnOff : Inport  Port=4
  Enable : EnablePort
  AND : Logic  AllPortsSameDT=off  OutDataTypeStr=boolean
  Compare To Constant1 : simulink/Logic and Bit Operations/Compare To Constant  relop===  const=BehindVeh_Detect  OutDataTypeStr=boolean
  Compare To Constant2 : simulink/Logic and Bit Operations/Compare To Constant  relop===  const=Ignition_ON  OutDataTypeStr=boolean
  Constant : Constant  Value=BrakeLightOn  SampleTime=-1
  Constant1 : Constant  Value=TailLightOn  SampleTime=-1
  Constant2 : Constant  Value=BrakeLightOff  SampleTime=-1
  OR : Logic  Operator=OR  AllPortsSameDT=off  OutDataTypeStr=boolean
  Switch : Switch  Criteria=u2 > Threshold  SaturateOnIntegerOverflow=off  InputSameDT=off
  Switch1 : Switch  Criteria=u2 > Threshold  SaturateOnIntegerOverflow=off  InputSameDT=off
  BrakeLight_IgnOn : Outport
  wires:
  Switch/1 -> BrakeLight_IgnOn/1
  Darkness/1 -> [Darkness]
  Veh_Detect/1 -> [Veh_Detect]
  Brake/1 -> AND/2
  IgnOnOff/1 -> Compare To Constant2/1
  OR/1 -> Switch/2
  Constant1/1 -> Switch1/1
  Constant/1 -> Switch/1
  [Veh_Detect] -> Compare To Constant1/1
  AND/1 -> OR/1
  Compare To Constant1/1 -> AND/1
  Constant2/1 -> Switch1/3
  Switch1/1 -> Switch/3
  [Darkness] -> OR/2
  Compare To Constant2/1 -> Switch1/2

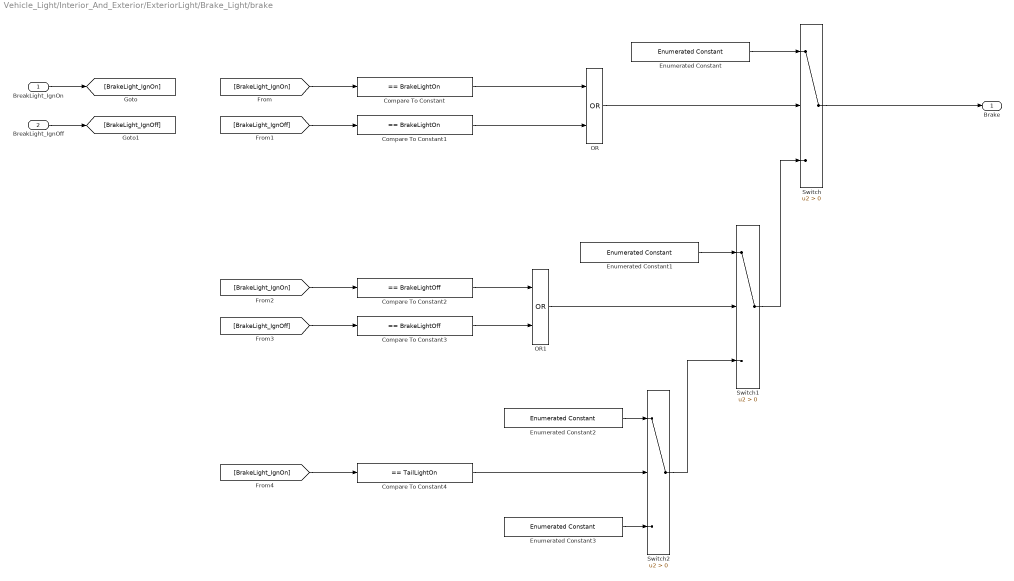
== system Vehicle_Light/Interior_And_Exterior/ExteriorLight/Brake_Light/brake ==
  BreakLight_IgnOn : Inport
  BreakLight_IgnOff : Inport  Port=2
  Compare To Constant : simulink/Logic and Bit Operations/Compare To Constant  relop===  const=BrakeLightOn  OutDataTypeStr=boolean
  Compare To Constant1 : simulink/Logic and Bit Operations/Compare To Constant  relop===  const=BrakeLightOn  OutDataTypeStr=boolean
  Compare To Constant2 : simulink/Logic and Bit Operations/Compare To Constant  relop===  const=BrakeLightOff  OutDataTypeStr=boolean
  Compare To Constant3 : simulink/Logic and Bit Operations/Compare To Constant  relop===  const=BrakeLightOff  OutDataTypeStr=boolean
  Compare To Constant4 : simulink/Logic and Bit Operations/Compare To Constant  relop===  const=TailLightOn  OutDataTypeStr=boolean
  Enumerated Constant : simulink/Sources/Enumerated Constant  OutDataTypeStr=Enum: LightSystem  Value=LightSystem.BrakeLightOn  SampleTime=-1
  Enumerated Constant1 : simulink/Sources/Enumerated Constant  OutDataTypeStr=Enum: LightSystem  Value=LightSystem.BrakeLightOff  SampleTime=-1
  Enumerated Constant2 : simulink/Sources/Enumerated Constant  OutDataTypeStr=Enum: LightSystem  Value=LightSystem.TailLightOn  SampleTime=-1
  Enumerated Constant3 : simulink/Sources/Enumerated Constant  OutDataTypeStr=Enum: LightSystem  Value=LightSystem.TailLightOff  SampleTime=-1
  OR : Logic  Operator=OR  AllPortsSameDT=off  OutDataTypeStr=boolean
  OR1 : Logic  Operator=OR  AllPortsSameDT=off  OutDataTypeStr=boolean
  Switch : Switch  Criteria=u2 > Threshold  SaturateOnIntegerOverflow=off  InputSameDT=off
  Switch1 : Switch  Criteria=u2 > Threshold  SaturateOnIntegerOverflow=off  InputSameDT=off
  Switch2 : Switch  Criteria=u2 > Threshold  SaturateOnIntegerOverflow=off  InputSameDT=off
  Brake : Outport
  wires:
  Switch/1 -> Brake/1
  Switch1/1 -> Switch/3
  OR/1 -> Switch/2
  BreakLight_IgnOn/1 -> [BrakeLight_IgnOn]
  [BrakeLight_IgnOn] -> Compare To Constant/1
  Compare To Constant/1 -> OR/1
  Compare To Constant1/1 -> OR/2
  BreakLight_IgnOff/1 -> [BrakeLight_IgnOff]
  [BrakeLight_IgnOff] -> Compare To Constant1/1
  [BrakeLight_IgnOff] -> Compare To Constant3/1
  Compare To Constant3/1 -> OR1/2
  Compare To Constant2/1 -> OR1/1
  [BrakeLight_IgnOn] -> Compare To Constant2/1
  OR1/1 -> Switch1/2
  Enumerated Constant/1 -> Switch/1
  Enumerated Constant1/1 -> Switch1/1
  Switch2/1 -> Switch1/3
  [BrakeLight_IgnOn] -> Compare To Constant4/1
  Compare To Constant4/1 -> Switch2/2
  Enumerated Constant2/1 -> Switch2/1
  Enumerated Constant3/1 -> Switch2/3

== system Vehicle_Light/Interior_And_Exterior/ExteriorLight/HeadLight/EscortLight_Veh_Lck_Unlock ==
  Darkness : Inport
  Key_Fob : Inport  Port=2
  VehicleLck : Inport  Port=3
  Enable : EnablePort
  escortLight_Veh_Lck_Unlock : Stateflow chart  TreatAsAtomicUnit=on
  EscortLight_Veh_Lck_Unlock : Outport
  wires:
  VehicleLck/1 -> escortLight_Veh_Lck_Unlock/3(VehicleLck)
  escortLight_Veh_Lck_Unlock/1(EscortLight) -> EscortLight_Veh_Lck_Unlock/1
  Darkness/1 -> escortLight_Veh_Lck_Unlock/1(Darkness)
  Key_Fob/1 -> escortLight_Veh_Lck_Unlock/2(Key_Fob)

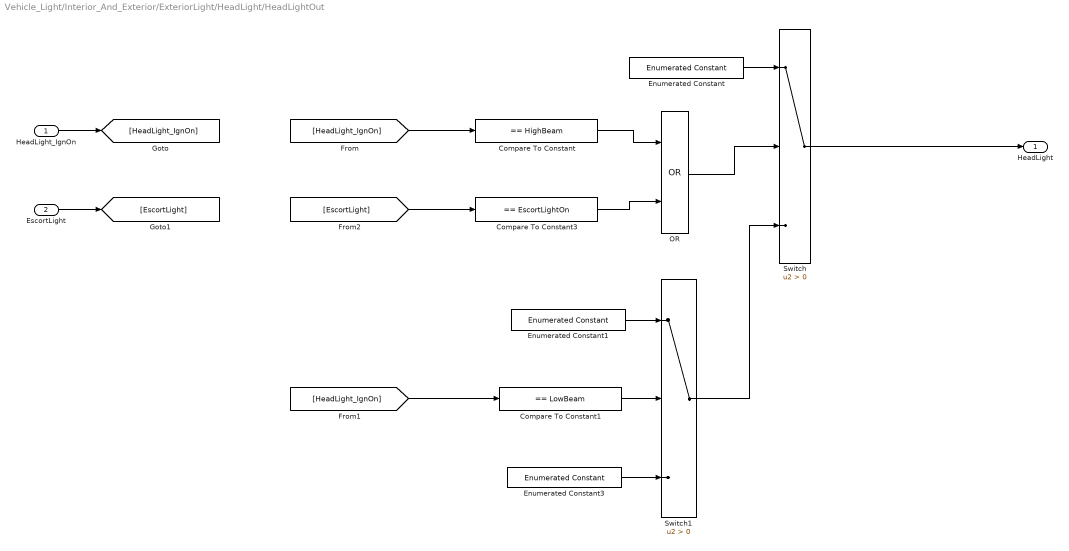
== system Vehicle_Light/Interior_And_Exterior/ExteriorLight/HeadLight/HeadLightOut ==
  HeadLight_IgnOn : Inport
  EscortLight : Inport  Port=2
  Compare To Constant : simulink/Logic and Bit Operations/Compare To Constant  relop===  const=HighBeam  OutDataTypeStr=boolean
  Compare To Constant1 : simulink/Logic and Bit Operations/Compare To Constant  relop===  const=LowBeam  OutDataTypeStr=boolean
  Compare To Constant3 : simulink/Logic and Bit Operations/Compare To Constant  relop===  const=EscortLightOn  OutDataTypeStr=boolean
  Enumerated Constant : simulink/Sources/Enumerated Constant  OutDataTypeStr=Enum: LightSystem  Value=LightSystem.HighBeam  SampleTime=-1
  Enumerated Constant1 : simulink/Sources/Enumerated Constant  OutDataTypeStr=Enum: LightSystem  Value=LightSystem.LowBeam  SampleTime=-1
  Enumerated Constant3 : simulink/Sources/Enumerated Constant  OutDataTypeStr=Enum: LightSystem  Value=LightSystem.HeadLightOff  SampleTime=-1
  OR : Logic  Operator=OR  AllPortsSameDT=off  OutDataTypeStr=boolean
  Switch : Switch  Criteria=u2 > Threshold  SaturateOnIntegerOverflow=off  InputSameDT=off
  Switch1 : Switch  Criteria=u2 > Threshold  SaturateOnIntegerOverflow=off  InputSameDT=off
  HeadLight : Outport
  wires:
  Enumerated Constant/1 -> Switch/1
  HeadLight_IgnOn/1 -> [HeadLight_IgnOn]
  [HeadLight_IgnOn] -> Compare To Constant/1
  Switch1/1 -> Switch/3
  Compare To Constant1/1 -> Switch1/2
  [HeadLight_IgnOn] -> Compare To Constant1/1
  Enumerated Constant1/1 -> Switch1/1
  Switch/1 -> HeadLight/1
  Enumerated Constant3/1 -> Switch1/3
  OR/1 -> Switch/2
  Compare To Constant/1 -> OR/1
  EscortLight/1 -> [EscortLight]
  [EscortLight] -> Compare To Constant3/1
  Compare To Constant3/1 -> OR/2

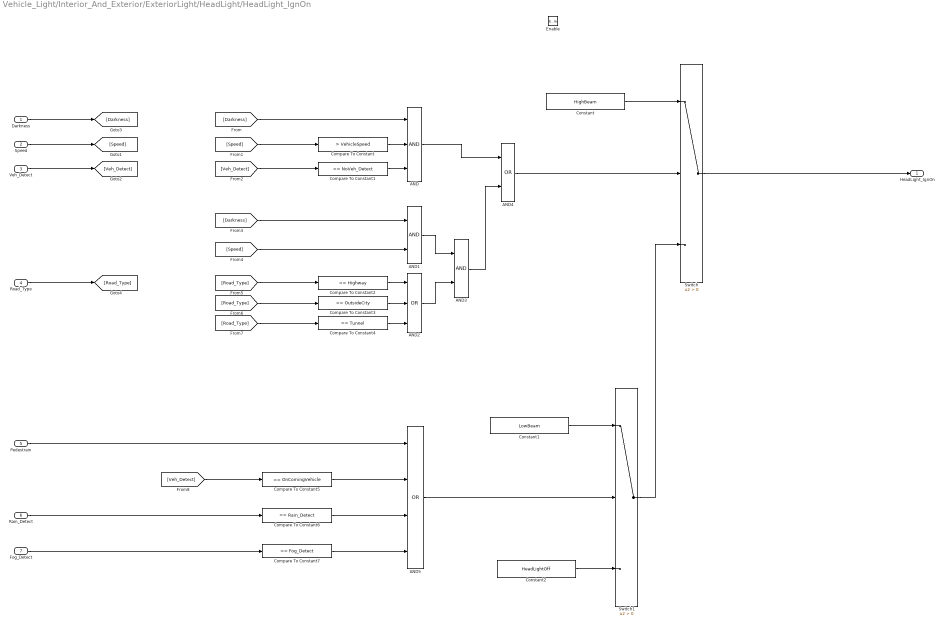
== system Vehicle_Light/Interior_And_Exterior/ExteriorLight/HeadLight/HeadLight_IgnOn ==
  Darkness : Inport
  Speed : Inport  Port=2
  Veh_Detect : Inport  Port=3
  Road_Type : Inport  Port=4
  Pedestrain : Inport  Port=5
  Rain_Detect : Inport  Port=6
  Fog_Detect : Inport  Port=7
  Enable : EnablePort
  AND : Logic  Inputs=3  AllPortsSameDT=off  OutDataTypeStr=boolean
  AND1 : Logic  AllPortsSameDT=off  OutDataTypeStr=boolean
  AND2 : Logic  Operator=OR  Inputs=3  AllPortsSameDT=off  OutDataTypeStr=boolean
  AND3 : Logic  AllPortsSameDT=off  OutDataTypeStr=boolean
  AND4 : Logic  Operator=OR  AllPortsSameDT=off  OutDataTypeStr=boolean
  AND5 : Logic  Operator=OR  Inputs=4  AllPortsSameDT=off  OutDataTypeStr=boolean
  Compare To Constant : simulink/Logic and Bit Operations/Compare To Constant  relop=>  const=VehicleSpeed  OutDataTypeStr=boolean
  Compare To Constant1 : simulink/Logic and Bit Operations/Compare To Constant  relop===  const=NoVeh_Detect  OutDataTypeStr=boolean
  Compare To Constant2 : simulink/Logic and Bit Operations/Compare To Constant  relop===  const=Highway  OutDataTypeStr=boolean
  Compare To Constant3 : simulink/Logic and Bit Operations/Compare To Constant  relop===  const=OutsideCity  OutDataTypeStr=boolean
  Compare To Constant4 : simulink/Logic and Bit Operations/Compare To Constant  relop===  const=Tunnel  OutDataTypeStr=boolean
  Compare To Constant5 : simulink/Logic and Bit Operations/Compare To Constant  relop===  const=OnComingVehicle  OutDataTypeStr=boolean
  Compare To Constant6 : simulink/Logic and Bit Operations/Compare To Constant  relop===  const=Rain_Detect  OutDataTypeStr=boolean
  Compare To Constant7 : simulink/Logic and Bit Operations/Compare To Constant  relop===  const=Fog_Detect  OutDataTypeStr=boolean
  Constant : Constant  Value=HighBeam  SampleTime=-1
  Constant1 : Constant  Value=LowBeam  SampleTime=-1
  Constant2 : Constant  Value=HeadLightOff  SampleTime=-1
  Switch : Switch  Criteria=u2 > Threshold  SaturateOnIntegerOverflow=off  InputSameDT=off
  Switch1 : Switch  Criteria=u2 > Threshold  SaturateOnIntegerOverflow=off  InputSameDT=off
  HeadLight_IgnOn : Outport
  wires:
  [Speed] -> Compare To Constant/1
  Veh_Detect/1 -> [Veh_Detect]
  [Road_Type] -> Compare To Constant3/1
  Speed/1 -> [Speed]
  Switch/1 -> HeadLight_IgnOn/1
  Constant2/1 -> Switch1/3
  [Speed] -> AND1/2
  Road_Type/1 -> [Road_Type]
  Compare To Constant4/1 -> AND2/3
  [Veh_Detect] -> Compare To Constant5/1
  [Darkness] -> AND1/1
  Compare To Constant2/1 -> AND2/1
  Constant/1 -> Switch/1
  Constant1/1 -> Switch1/1
  Fog_Detect/1 -> Compare To Constant7/1
  Compare To Constant1/1 -> AND/3
  Compare To Constant/1 -> AND/2
  Rain_Detect/1 -> Compare To Constant6/1
  [Veh_Detect] -> Compare To Constant1/1
  Compare To Constant5/1 -> AND5/2
  Pedestrain/1 -> AND5/1
  AND5/1 -> Switch1/2
  AND4/1 -> Switch/2
  [Road_Type] -> Compare To Constant2/1
  Compare To Constant3/1 -> AND2/2
  AND1/1 -> AND3/1
  AND2/1 -> AND3/2
  [Darkness] -> AND/1
  AND3/1 -> AND4/2
  Switch1/1 -> Switch/3
  Compare To Constant7/1 -> AND5/4
  AND/1 -> AND4/1
  Darkness/1 -> [Darkness]
  Compare To Constant6/1 -> AND5/3
  [Road_Type] -> Compare To Constant4/1

== system Vehicle_Light/Interior_And_Exterior/ExteriorLight/hazardLight/HazardLightIgnOff ==
  Darkness : Inport
  Veh_Position : Inport  Port=2
  Enable : EnablePort
  HazardLight : Stateflow chart  TreatAsAtomicUnit=on
  HazardLightOff : Outport
  wires:
  HazardLight/1(HazardLight) -> HazardLightOff/1
  Darkness/1 -> HazardLight/1(Darkness)
  Veh_Position/1 -> HazardLight/2(Veh_Position)

== system Vehicle_Light/Interior_And_Exterior/ExteriorLight/hazardLight/HazardLightIgnOn ==
  Darkness : Inport
  Veh_Position : Inport  Port=2
  Enable : EnablePort
  AND : Logic  AllPortsSameDT=off  OutDataTypeStr=boolean
  Compare To Constant : simulink/Logic and Bit Operations/Compare To Constant  relop===  const=StationaryPosition  OutDataTypeStr=boolean
  Compare To Constant1 : simulink/Logic and Bit Operations/Compare To Constant  relop===  const=BrokeDownPosition  OutDataTypeStr=boolean
  Constant : Constant  Value=HazardLightOff  SampleTime=-1
  Constant1 : Constant  Value=HazardLightOn  SampleTime=-1
  Constant2 : Constant  Value=HazardLightOn  SampleTime=-1
  Switch : Switch  Criteria=u2 > Threshold  SaturateOnIntegerOverflow=off  InputSameDT=off
  Switch1 : Switch  Criteria=u2 > Threshold  SaturateOnIntegerOverflow=off  InputSameDT=off
  HazardLightOn : Outport
  wires:
  Switch1/1 -> Switch/3
  Constant1/1 -> Switch/1
  AND/1 -> Switch/2
  Veh_Position/1 -> [Veh_Position]
  [Veh_Position] -> Compare To Constant1/1
  Constant2/1 -> Switch1/1
  Compare To Constant1/1 -> Switch1/2
  [Veh_Position] -> Compare To Constant/1
  Constant/1 -> Switch1/3
  Compare To Constant/1 -> AND/2
  Darkness/1 -> AND/1
  Switch/1 -> HazardLightOn/1

== system Vehicle_Light/Interior_And_Exterior/ExteriorLight/hazardLight/Subsystem ==
  HazardLightIgnOn : Inport
  HazardLightIgnOff : Inport  Port=2
  Compare To Constant : simulink/Logic and Bit Operations/Compare To Constant  relop===  const=HazardLightOn  OutDataTypeStr=boolean
  Compare To Constant1 : simulink/Logic and Bit Operations/Compare To Constant  relop===  const=HazardLightOn  OutDataTypeStr=boolean
  Enumerated Constant : simulink/Sources/Enumerated Constant  OutDataTypeStr=Enum: LightSystem  Value=LightSystem.HazardLightOn  SampleTime=-1
  Enumerated Constant1 : simulink/Sources/Enumerated Constant  OutDataTypeStr=Enum: LightSystem  Value=LightSystem.HazardLightOff  SampleTime=-1
  OR : Logic  Operator=OR  AllPortsSameDT=off  OutDataTypeStr=boolean
  Switch : Switch  Criteria=u2 > Threshold  SaturateOnIntegerOverflow=off  InputSameDT=off
  Hazard : Outport
  wires:
  Switch/1 -> Hazard/1
  OR/1 -> Switch/2
  HazardLightIgnOn/1 -> [HazardLightIgnOn]
  HazardLightIgnOff/1 -> [HazardLightIgnOff]
  Compare To Constant/1 -> OR/1
  [HazardLightIgnOn] -> Compare To Constant/1
  Compare To Constant1/1 -> OR/2
  [HazardLightIgnOff] -> Compare To Constant1/1
  Enumerated Constant/1 -> Switch/1
  Enumerated Constant1/1 -> Switch/3

== system Vehicle_Light/Interior_And_Exterior/ExteriorLight/indicatorLight/Subsystem ==
  IndicatorLight : Inport
  Compare To Constant : simulink/Logic and Bit Operations/Compare To Constant  relop===  const=RightIndicator  OutDataTypeStr=boolean
  Compare To Constant1 : simulink/Logic and Bit Operations/Compare To Constant  relop===  const=LeftIndicator  OutDataTypeStr=boolean
  Enumerated Constant : simulink/Sources/Enumerated Constant  OutDataTypeStr=Enum: LightSystem  Value=LightSystem.RightIndicatorOn  SampleTime=inf
  Enumerated Constant1 : simulink/Sources/Enumerated Constant  OutDataTypeStr=Enum: LightSystem  Value=LightSystem.LeftIndicatorOn  SampleTime=inf
  Enumerated Constant2 : simulink/Sources/Enumerated Constant  OutDataTypeStr=Enum: LightSystem  Value=LightSystem.IndicatorOff  SampleTime=inf
  Switch : Switch  Criteria=u2 > Threshold  SaturateOnIntegerOverflow=off  InputSameDT=off
  Switch1 : Switch  Criteria=u2 > Threshold  SaturateOnIntegerOverflow=off  InputSameDT=off
  IndicatorLightOnOFF : Outport
  wires:
  Switch/1 -> IndicatorLightOnOFF/1
  Compare To Constant/1 -> Switch/2
  Switch1/1 -> Switch/3
  Compare To Constant1/1 -> Switch1/2
  Enumerated Constant/1 -> Switch/1
  Enumerated Constant1/1 -> Switch1/1
  Enumerated Constant2/1 -> Switch1/3
  [IndicatorLight] -> Compare To Constant/1
  [IndicatorLight] -> Compare To Constant1/1
  IndicatorLight/1 -> [IndicatorLight]

== system Vehicle_Light/Interior_And_Exterior/Interior_Light/readingLight/Subsystem ==
  Gesture_Detect : Inport
  Door : Inport  Port=2
  Enable : EnablePort
  Compare To Constant : simulink/Logic and Bit Operations/Compare To Constant  relop===  const=DoorOpen  OutDataTypeStr=boolean
  Constant : Constant  Value=ReadingLightOn  SampleTime=-1
  Constant1 : Constant  Value=ReadingLightOff  SampleTime=-1
  OR : Logic  Operator=OR  AllPortsSameDT=off  OutDataTypeStr=boolean
  Switch : Switch  Criteria=u2 > Threshold  SaturateOnIntegerOverflow=off  InputSameDT=off
  ReadingLight_IgnOn : Outport
  wires:
  Compare To Constant/1 -> OR/2
  Constant1/1 -> Switch/3
  OR/1 -> Switch/2
  Switch/1 -> ReadingLight_IgnOn/1
  Door/1 -> Compare To Constant/1
  Gesture_Detect/1 -> OR/1
  Constant/1 -> Switch/1

== system Vehicle_Light/Interior_And_Exterior/Interior_Light/readingLight/Subsystem1 ==
  VehicleLck : Inport
  Darkness : Inport  Port=2
  Key_Fob : Inport  Port=3
  Enable : EnablePort
  ReadingLight : Stateflow chart  TreatAsAtomicUnit=on
  ReadingLight_IgnOff : Outport
  wires:
  ReadingLight/1(ReadingLight) -> ReadingLight_IgnOff/1
  VehicleLck/1 -> ReadingLight/1(VehicleLck)
  Darkness/1 -> ReadingLight/2(Darkness)
  Key_Fob/1 -> ReadingLight/3(Key_Fob)

== system Vehicle_Light/Interior_And_Exterior/Interior_Light/readingLight/Subsystem2 ==
  ReadingLight_IgnOn : Inport
  ReadingLight_IgnOff : Inport  Port=2
  Compare To Constant : simulink/Logic and Bit Operations/Compare To Constant  relop===  const=ReadingLightOn  OutDataTypeStr=boolean
  Compare To Constant1 : simulink/Logic and Bit Operations/Compare To Constant  relop===  const=ReadingLightOn  OutDataTypeStr=boolean
  Enumerated Constant : simulink/Sources/Enumerated Constant  OutDataTypeStr=Enum: LightSystem  Value=LightSystem.ReadingLightOn  SampleTime=-1
  Enumerated Constant1 : simulink/Sources/Enumerated Constant  OutDataTypeStr=Enum: LightSystem  Value=LightSystem.ReadingLightOff  SampleTime=-1
  OR : Logic  Operator=OR  AllPortsSameDT=off  OutDataTypeStr=boolean
  Switch : Switch  Criteria=u2 > Threshold  SaturateOnIntegerOverflow=off  InputSameDT=off
  ReadingLight : Outport
  wires:
  OR/1 -> Switch/2
  Compare To Constant/1 -> OR/1
  ReadingLight_IgnOn/1 -> Compare To Constant/1
  Compare To Constant1/1 -> OR/2
  ReadingLight_IgnOff/1 -> Compare To Constant1/1
  Switch/1 -> ReadingLight/1
  Enumerated Constant/1 -> Switch/1
  Enumerated Constant1/1 -> Switch/3

== stateflow chart Vehicle_Light/Interior_And_Exterior/ExteriorLight/hazardLight/HazardLightIgnOff/HazardLight ==
  settings: executeAtInitialization=1
  state HazardOff
    en:
    HazardLight=0
  state HazardOn
    en:
    HazardLight=1
  state HazardOn_BreakDown_
    en:
    HazardLight=1
  (default) -> HazardOff
  HazardOff -> HazardOn [order 1] : [Veh_Position==0&&Darkness==1]
  HazardOn -> HazardOff [order 1] : after(5,sec)
  HazardOn -> HazardOff [order 3] : [Darkness==0]
  HazardOn -> HazardOn_BreakDown_ [order 2] : [ Veh_Position==1]
  HazardOn_BreakDown_ -> HazardOff : [Veh_Position~=1]
  HazardOff -> HazardOn_BreakDown_ [order 2] : [Veh_Position==1]
  data: Darkness input; Veh_Position input; HazardLight output

== stateflow chart Vehicle_Light/Interior_And_Exterior/ExteriorLight/indicatorLight/Indicator ==
  settings: executeAtInitialization=1
  state IndicatorON
    en:
    Indicator=1
  state IndicatorOff
    en:
    Indicator=0
  state IndicatorON1
    en:
    Indicator=2
  (default) -> IndicatorOff
  IndicatorOff -> IndicatorON [order 1] : [Steering_Angle>=10]
  IndicatorON -> IndicatorOff [order 2] : after(10,sec)[Steering_Angle<10]
  IndicatorON1 -> IndicatorON [order 2] : [Steering_Angle>=10]
  IndicatorON -> IndicatorON1 [order 1] : [Steering_Angle<=-10]
  IndicatorOff -> IndicatorON1 [order 2] : [Steering_Angle<=-10]
  IndicatorON1 -> IndicatorOff [order 1] : after(10,sec)[Steering_Angle>-10]
  data: Steering_Angle input; Indicator output

== stateflow chart Vehicle_Light/Interior_And_Exterior/ExteriorLight/HeadLight/EscortLight_Veh_Lck_Unlock/escortLight_Veh_Lck_Unlock ==
  settings: executeAtInitialization=1
  state EscortLight
    en:
    EscortLight=0
  state EscortLight1
    en:
    EscortLight=1
  (default) -> EscortLight
  EscortLight -> (junction 29) : [Darkness==1&&Key_Fob<=10]
  (junction 29) -> EscortLight1 : [VehicleLck==0||VehicleLck==1]
  EscortLight1 -> EscortLight : after(10,sec)[Darkness==0]
  data: Darkness input; Key_Fob input; VehicleLck input; EscortLight output

== stateflow chart Vehicle_Light/Interior_And_Exterior/Interior_Light/readingLight/Subsystem1/ReadingLight ==
  settings: executeAtInitialization=1
  state ReadingLight1
    en:
    ReadingLight=1
  state ReadingLight
    en:
    ReadingLight=0
  (default) -> ReadingLight
  ReadingLight -> (junction 20) : [VehicleLck==0||VehicleLck==1]
  (junction 20) -> (junction 22) : [Darkness==1]
  (junction 22) -> ReadingLight1 : [Key_Fob<=10]
  ReadingLight1 -> ReadingLight [order 2] : after(10,sec)
  ReadingLight1 -> ReadingLight [order 1] : [Darkness==0]
  data: VehicleLck input; ReadingLight output; Darkness input; Key_Fob input

== stateflow chart Vehicle_Light/Interior_And_Exterior/ExteriorLight/Brake_Light/BrakeLight_IgnOff/Chart1 ==
  settings: executeAtInitialization=1
  state Brake
    en:
    BrakeLight=0
  state Brake1
    en:
    BrakeLight=1
  (default) -> Brake
  Brake -> (junction 14) : [VehicleLck==0||VehicleLck==1]
  (junction 14) -> (junction 16) : [Darkness==1]
  (junction 16) -> Brake1 : [Key_Fob<=10]
  Brake1 -> Brake [order 1] : after(10,sec)
  Brake1 -> Brake [order 2] : [Darkness==0]
  data: BrakeLight output; VehicleLck input; Darkness input; Key_Fob input
